simulink model "Simulation_V_change"  (R2024a)
settings: Solver=VariableStepAuto  StartTime=0.0  StopTime=10.0  RelTol=1e-3
undefined symbols (not defined in the file or in its folder): Ts
libraries: spsThreePhaseSineGeneratorLib x1, spsPLL3phLib x1, spsPositiveSequencePLLDrivenLib x1
settings Model: Creator=E370_  LastModifiedBy=E370_

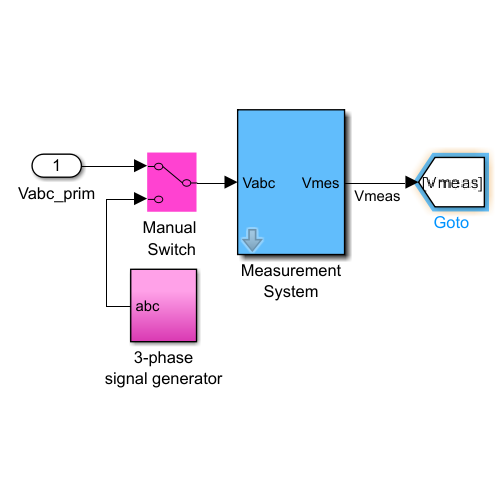
[thumbnail: Simulink's stored preview of the top-level diagram]
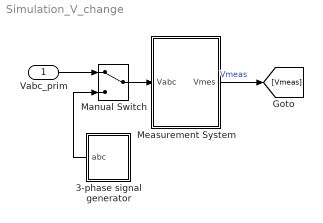
== system Simulation_V_change ==
  Vabc_prim : Inport  PortDimensions=3
  3-phase signal generator : Subsystem
  Manual Switch : ManualSwitch
  Measurement System : Subsystem  mask(SVC measurement system){Vnom=735e3, ParI=[735e3*0.9998 0 60], Ts=Ts}
      mask prompts: Vnom "Nominal voltage (volts rms ph-ph)"; ParI "Initial input: [ Mag (volts rms ph-ph)  Phase (degree) Freq (Hz) ]"; Ts "Sample time:"
      mask init:
      | Mag_Init=ParI(1)/Vnom;
      | Phase_Init=ParI(2);
      | Freq_Init=ParI(3);
  wires:
  Manual Switch/1 -> Measurement System/1(Vabc)
  3-phase signal generator/1(abc) -> Manual Switch/2
  Vabc_prim/1 -> Manual Switch/1
  Measurement System/1(Vmes) -> [Vmeas]  "Vmeas"

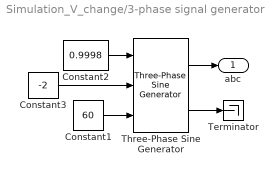
== system Simulation_V_change/3-phase signal generator ==
  Constant1 : Constant  Value=60
  Constant2 : Constant  Value=0.9998
  Constant3 : Constant  Value=-2
  Terminator : Terminator
  Three-Phase Sine Generator : spsThreePhaseSineGeneratorLib/Three-Phase Sine Generator  Ts=Ts
  abc : Outport  VectorParamsAs1DForOutWhenUnconnected=off
  wires:
  Constant1/1 -> Three-Phase Sine Generator/3
  Constant2/1 -> Three-Phase Sine Generator/1
  Constant3/1 -> Three-Phase Sine Generator/2
  Three-Phase Sine Generator/1 -> abc/1
  Three-Phase Sine Generator/2 -> Terminator/1

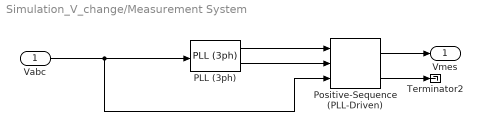
== system Simulation_V_change/Measurement System ==
  Vabc : Inport  PortDimensions=3
  PLL (3ph) : spsPLL3phLib/PLL (3ph)  Fmin=45  Par_Init=[Phase_Init Freq_Init]  ParK=[60 1400 0]  TcD=1e-4  MaxRateChangeFreq=12  FilterCutOffFreq=25  Ts=Ts  AGC=off
  Positive-Sequence (PLL-Driven) : spsPositiveSequencePLLDrivenLib/Positive-Sequence (PLL-Driven)  Finit=Freq_Init  Fmin=45  InInit=[Mag_Init 0]  Ts=Ts
  Terminator2 : Terminator
  Vmes : Outport  VectorParamsAs1DForOutWhenUnconnected=off
  wires:
  PLL (3ph)/1 -> Positive-Sequence (PLL-Driven)/1
  PLL (3ph)/2 -> Positive-Sequence (PLL-Driven)/2
  Vabc/1 -> Positive-Sequence (PLL-Driven)/3, PLL (3ph)/1
  Positive-Sequence (PLL-Driven)/2 -> Terminator2/1
  Positive-Sequence (PLL-Driven)/1 -> Vmes/1
